simulink model "fcn2"  (R2017b)
settings: Solver=VariableStepAuto  StartTime=0.0  StopTime=10.0  RelTol=1e-3
settings Model: Creator=ghleila  LastModifiedBy=ghleila

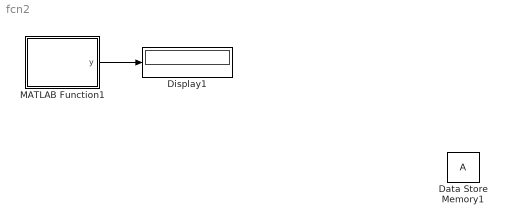
== system fcn2 ==
  Data Store Memory1 : DataStoreMemory  InitialValue=30  ShowAdditionalParam=off  OutDataTypeStr=double
  Display1 : Display
  MATLAB Function1 : MATLAB Function  TreatAsAtomicUnit=on
  wires:
  MATLAB Function1/1(y) -> Display1/1

== matlab function fcn2/MATLAB Function1 ==
  data: y output; A data_store_memory
function y = fcn
%#codegen
global H;
H = H+1;
y = H;
